simulink model "Temp"  (R2021a)
settings: Solver=FixedStepAuto  StartTime=0.0  StopTime=10.0  FixedStep=1e-3  RelTol=1e-3  EnableMultiTasking=on
undefined symbols (not defined in the file): D0, D10, D11, D12, D13, D2, D4, D5, D6, D7, D8, D9, PTA0, PTA2, PTB23, PTB9, PTC16, PTC2, PTC3, PTC4, PTD0, PTD1, PTD2, PTD3
libraries: frdmk64flib x16
settings Model: PacingRate=0.250000  ExtModeTrigDuration=5  Creator=Arun Mistry  LastModifiedBy=Arun Mistry
settings OptimizationCC: EnhancedBackFolding=on  PassReuseOutputArgsAs=Individual arguments  ZeroExternalMemoryAtStartup=off  ZeroInternalMemoryAtStartup=off  MaxStackSize=64  OptimizeBlockOrder=speed  DifferentSizesBufferReuse=on  OptimizationCustomize=off  EfficientTunableParamExpr=on
settings DebuggingCC: ParameterTunabilityLossMsg=error
settings HardwareCC: ProdBitPerPointer=32  ProdBitPerSizeT=32  ProdBitPerPtrDiffT=32  ProdLargestAtomicInteger=Long  ProdLargestAtomicFloat=Double  ProdWordSize=32  ProdHWDeviceType=ARM Compatible->ARM Cortex
settings SFSimCC: MATLABDynamicMemAlloc=off
settings RTWCC: SystemTargetFile=ert.tlc  HardwareBoard=NXP FRDM-K64F  TLCOptions="-aInlineSetEventsForThisBaseRateFcn=TLC_FALSE -aSuppressMultiTaskScheduler=TLC_FALSE  -aRateBasedStepFcn=0"  TemplateMakefile=ert_default_tmf  Toolchain=GNU Tools for ARM Embedded Processors
settings CodeAppCC: ForceParamTrailComments=on  IgnoreCustomStorageClasses=off  OperatorAnnotations=on  SimulinkDataObjDesc=on  SFDataObjDesc=on  InsertBlockDesc=on
settings ERTTargetCC: ExtModeTransport=4  ExtModeMexFile=sendToCommService

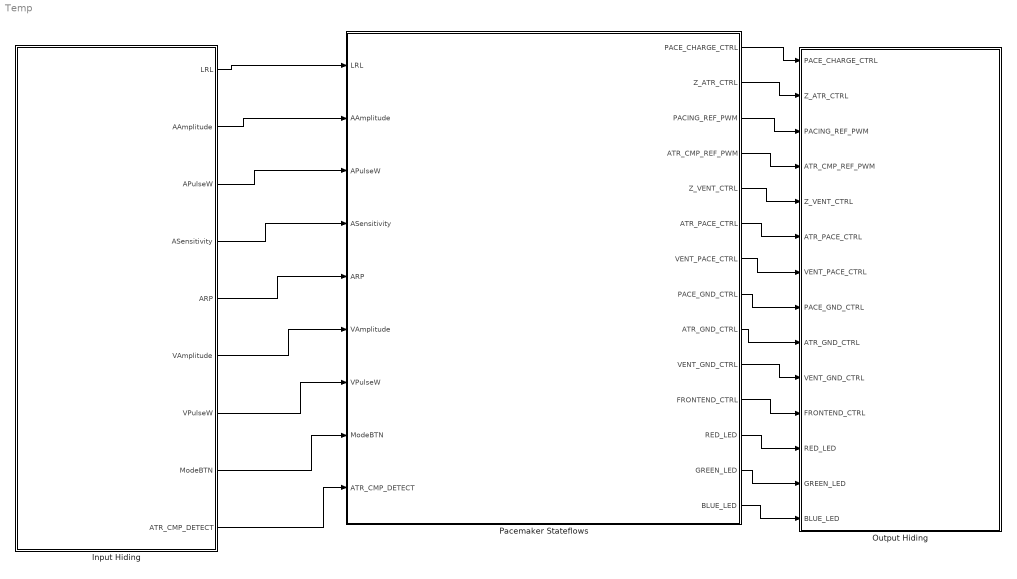
== system Temp ==
  Input Hiding : Subsystem
  Output Hiding : Subsystem
  Pacemaker Stateflows : Stateflow chart  TreatAsAtomicUnit=on
      settings: PortSchema="{\"entries\":[{\"content\":{\"sides\":[{\"content\":{\"connectorIds\":[\"In1\",\"In2\",\"In4\",\"In3\",\"In5\",\"In6\",\"In7\",\"In8\",\"In9\"]},\"type\":\"ConnectorPlacement.EquallySpacedRectSide\",\"uuid\":\"2299fccd-18a7-4758-b9fd-98bed0ea2d5f\"},{\"content\":{\"connectorIds\":[\"Out1\",\"Out2\",\"Out3\",\"Out4\",\"Out5\",\"Out6\",\"Out7\",\"Out8\",\"Out9\",\"Out10\",\"Out11\",\"Out12\",\"Out13\",\"Out14\"],\"side\":\"RIGHT\"},\"type\":\"ConnectorPlacement.EquallySpacedRectSide\",\"uuid\":\"a580a96d-c680-40ce-9bea-87ad4b87457c\"},{\"content\":{\"connectorIds\":[],\"side\":\"TOP\"},\"type\":\"ConnectorPlacement.EquallySpacedRectSide\",\"uuid\":\"b356f760-e5f1-4f6b-abb2-2757fd914320\"}]},\"type\":\"ConnectorPlacement.EquallySpacedConnector\",\"uuid\":\"b29a7396-67ba-49d5-b173-a751f9e05efc\"}],\"packageUris\":[\"http://schema.mathworks.com/mf0/Connector/R2020b\"],\"version\":\"1.0\"}"
  wires:
  Input Hiding/8(ModeBTN) -> Pacemaker Stateflows/8(ModeBTN)
  Input Hiding/2(AAmplitude) -> Pacemaker Stateflows/2(AAmplitude)
  Pacemaker Stateflows/2(Z_ATR_CTRL) -> Output Hiding/2(Z_ATR_CTRL)
  Pacemaker Stateflows/9(ATR_GND_CTRL) -> Output Hiding/9(ATR_GND_CTRL)
  Input Hiding/6(VAmplitude) -> Pacemaker Stateflows/6(VAmplitude)
  Pacemaker Stateflows/6(ATR_PACE_CTRL) -> Output Hiding/6(ATR_PACE_CTRL)
  Input Hiding/3(APulseW) -> Pacemaker Stateflows/4(APulseW)
  Pacemaker Stateflows/5(Z_VENT_CTRL) -> Output Hiding/5(Z_VENT_CTRL)
  Pacemaker Stateflows/3(PACING_REF_PWM) -> Output Hiding/3(PACING_REF_PWM)
  Pacemaker Stateflows/10(VENT_GND_CTRL) -> Output Hiding/10(VENT_GND_CTRL)
  Pacemaker Stateflows/8(PACE_GND_CTRL) -> Output Hiding/8(PACE_GND_CTRL)
  Pacemaker Stateflows/7(VENT_PACE_CTRL) -> Output Hiding/7(VENT_PACE_CTRL)
  Input Hiding/1(LRL) -> Pacemaker Stateflows/1(LRL)
  Input Hiding/7(VPulseW) -> Pacemaker Stateflows/7(VPulseW)
  Pacemaker Stateflows/1(PACE_CHARGE_CTRL) -> Output Hiding/1(PACE_CHARGE_CTRL)
  Input Hiding/4(ASensitivity) -> Pacemaker Stateflows/3(ASensitivity)
  Input Hiding/5(ARP) -> Pacemaker Stateflows/5(ARP)
  Input Hiding/9(ATR_CMP_DETECT) -> Pacemaker Stateflows/9(ATR_CMP_DETECT)
  Pacemaker Stateflows/12(RED_LED) -> Output Hiding/12(RED_LED)
  Pacemaker Stateflows/13(GREEN_LED) -> Output Hiding/13(GREEN_LED)
  Pacemaker Stateflows/11(FRONTEND_CTRL) -> Output Hiding/11(FRONTEND_CTRL)
  Pacemaker Stateflows/4(ATR_CMP_REF_PWM) -> Output Hiding/4(ATR_CMP_REF_PWM)
  Pacemaker Stateflows/14(BLUE_LED) -> Output Hiding/14(BLUE_LED)

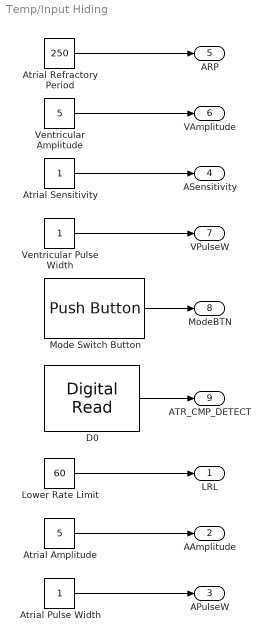
== system Temp/Input Hiding ==
  Atrial Amplitude : Constant  Value=5  OutDataTypeStr=double
  Atrial Pulse Width : Constant  OutDataTypeStr=double
  Atrial Refractory Period : Constant  Value=250  OutDataTypeStr=double
  Atrial Sensitivity : Constant  OutDataTypeStr=double
  D0 : frdmk64flib/Digital Read  Whichpin=PTC16 (D0)  SampleTime=-1
  Lower Rate Limit : Constant  Value=60  OutDataTypeStr=double
  Mode Switch Button : frdmk64flib/Push Button  Whichswitch=SW2  SampleTime1=-1
  Ventricular Amplitude : Constant  Value=5  OutDataTypeStr=double
  Ventricular Pulse Width : Constant  OutDataTypeStr=double
  LRL : Outport  OutDataTypeStr=double
  AAmplitude : Outport  Port=2  OutDataTypeStr=double
  APulseW : Outport  Port=3  OutDataTypeStr=double
  ASensitivity : Outport  Port=4  OutDataTypeStr=double
  ARP : Outport  Port=5  OutDataTypeStr=double
  VAmplitude : Outport  Port=6  OutDataTypeStr=double
  VPulseW : Outport  Port=7  OutDataTypeStr=double
  ModeBTN : Outport  Port=8  OutDataTypeStr=boolean
  ATR_CMP_DETECT : Outport  Port=9  OutDataTypeStr=boolean
  wires:
  Ventricular Amplitude/1 -> VAmplitude/1
  Mode Switch Button/1 -> ModeBTN/1
  D0/1 -> ATR_CMP_DETECT/1
  Atrial Refractory Period/1 -> ARP/1
  Ventricular Pulse Width/1 -> VPulseW/1
  Atrial Sensitivity/1 -> ASensitivity/1
  Atrial Pulse Width/1 -> APulseW/1
  Atrial Amplitude/1 -> AAmplitude/1
  Lower Rate Limit/1 -> LRL/1

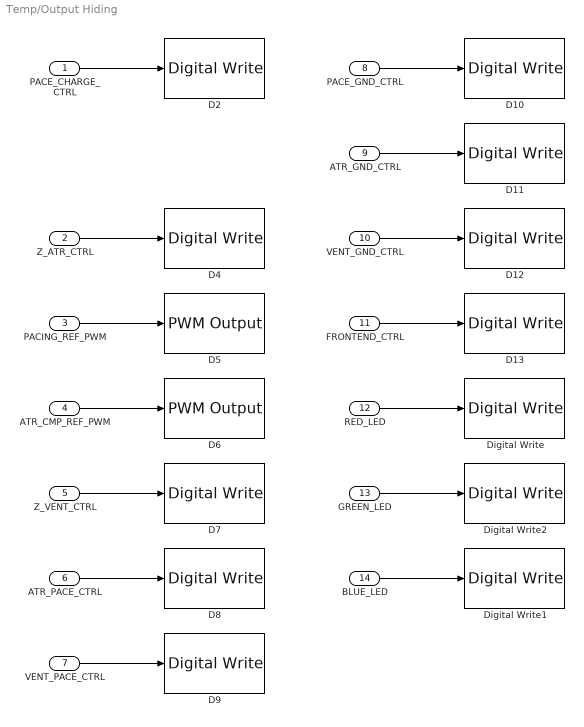
== system Temp/Output Hiding ==
  PACE_CHARGE_CTRL : Inport  OutDataTypeStr=double
  Z_ATR_CTRL : Inport  Port=2  OutDataTypeStr=double
  PACING_REF_PWM : Inport  Port=3  OutDataTypeStr=double
  ATR_CMP_REF_PWM : Inport  Port=4  OutDataTypeStr=double
  Z_VENT_CTRL : Inport  Port=5  OutDataTypeStr=double
  ATR_PACE_CTRL : Inport  Port=6  OutDataTypeStr=double
  VENT_PACE_CTRL : Inport  Port=7  OutDataTypeStr=double
  PACE_GND_CTRL : Inport  Port=8  OutDataTypeStr=double
  ATR_GND_CTRL : Inport  Port=9  OutDataTypeStr=double
  VENT_GND_CTRL : Inport  Port=10  OutDataTypeStr=double
  FRONTEND_CTRL : Inport  Port=11  OutDataTypeStr=double
  RED_LED : Inport  Port=12  OutDataTypeStr=double
  GREEN_LED : Inport  Port=13  OutDataTypeStr=double
  BLUE_LED : Inport  Port=14  OutDataTypeStr=double
  D10 : frdmk64flib/Digital Write  Whichpin=PTD0 (D10)
  D11 : frdmk64flib/Digital Write  Whichpin=PTD2 (D11)
  D12 : frdmk64flib/Digital Write  Whichpin=PTD3 (D12)
  D13 : frdmk64flib/Digital Write  Whichpin=PTD1 (D13)
  D2 : frdmk64flib/Digital Write  Whichpin=PTB9 (D2)
  D4 : frdmk64flib/Digital Write  Whichpin=PTB23 (D4)
  D5 : frdmk64flib/PWM Output  Whichpin=PTA2 (D5)  InitialFrequency=2000  InitialDutyCycle=100
  D6 : frdmk64flib/PWM Output  Whichpin=PTC2 (D6)  InitialFrequency=916  InitialDutyCycle=0
  D7 : frdmk64flib/Digital Write  Whichpin=PTC3 (D7)
  "D8 " : frdmk64flib/Digital Write  Whichpin=PTA0 (D8)
  D9 : frdmk64flib/Digital Write  Whichpin=PTC4 (D9)
  Digital Write : frdmk64flib/Digital Write  Whichpin=RED_LED
  Digital Write1 : frdmk64flib/Digital Write  Whichpin=BLUE_LED
  Digital Write2 : frdmk64flib/Digital Write  Whichpin=GREEN_LED
  wires:
  VENT_PACE_CTRL/1 -> D9/1
  ATR_CMP_REF_PWM/1 -> D6/1
  PACE_GND_CTRL/1 -> D10/1
  PACING_REF_PWM/1 -> D5/1
  ATR_GND_CTRL/1 -> D11/1
  ATR_PACE_CTRL/1 -> "D8 "/1
  PACE_CHARGE_CTRL/1 -> D2/1
  FRONTEND_CTRL/1 -> D13/1
  VENT_GND_CTRL/1 -> D12/1
  Z_ATR_CTRL/1 -> D4/1
  Z_VENT_CTRL/1 -> D7/1
  RED_LED/1 -> Digital Write/1
  GREEN_LED/1 -> Digital Write2/1
  BLUE_LED/1 -> Digital Write1/1

== stateflow chart Temp/Pacemaker Stateflows ==
  state AOO
    state ENTRY
      entry:
      VENT_PACE_CTRL = 0; VENT_GND_CTRL = 0; PACE_GND_CTRL = 1;
      Z_VENT_CTRL = 0; Z_ATR_CTRL = 0; PACING_REF_PWM = AAmplitude*20;
    state PACE_ATR
      entry:
      PACE_CHARGE_CTRL = 0;
      ATR_GND_CTRL = 0;
      ATR_PACE_CTRL = 1;
      RED_LED = 1;
    state C22_CHARGE
      entry:
      ATR_PACE_CTRL = 0;
      ATR_GND_CTRL = 1;
      PACE_CHARGE_CTRL = 1;
      RED_LED = 0;
    (default) -> AOO.ENTRY
    AOO.ENTRY -> AOO.C22_CHARGE
    AOO.PACE_ATR -> AOO.C22_CHARGE : after(APulseW,msec)
    AOO.C22_CHARGE -> AOO.PACE_ATR : after((60000/LRL)-APulseW,msec)
  state VOO
    state ENTRY
      entry:
      ATR_PACE_CTRL = 0; ATR_GND_CTRL = 0; PACE_GND_CTRL = 1;
      Z_ATR_CTRL = 0; Z_VENT_CTRL = 0; PACING_REF_PWM = VAmplitude*20;
    state PACE_VENT
      entry:
      PACE_CHARGE_CTRL = 0;
      VENT_GND_CTRL = 0;
      VENT_PACE_CTRL = 1;
      BLUE_LED = 1;
    state C22_CHARGE
      entry:
      VENT_PACE_CTRL = 0;
      VENT_GND_CTRL = 1;
      PACE_CHARGE_CTRL = 1;
      BLUE_LED = 0;
    (default) -> VOO.ENTRY
    VOO.ENTRY -> VOO.C22_CHARGE
    PACE_VENT -> VOO.C22_CHARGE : after(VPulseW,msec)
    VOO.C22_CHARGE -> PACE_VENT : after((60000/LRL)-VPulseW,msec)
  state MODE
    entry:
    Mode = Mode + 1;
    Mode = rem(Mode ,4);
  state AAI
    state ENTRY
      entry:
      VENT_PACE_CTRL = 0; VENT_GND_CTRL = 0; PACE_GND_CTRL = 1;
      Z_VENT_CTRL = 0; Z_ATR_CTRL = 0; PACING_REF_PWM = AAmplitude*20;
      FRONTEND_CTRL = 1;
    state PACE_ATR
      %Discharge
      entry:
      PACE_CHARGE_CTRL = 0;
      ATR_GND_CTRL = 0;
      ATR_PACE_CTRL = 1;
    state C22_CHARGE
      entry:
      ATR_PACE_CTRL = 0;
      ATR_GND_CTRL = 1;
      PACE_CHARGE_CTRL = 1;
    state INTERMEDIATE
      %In between state
      entry:
      PACE_CHARGE_CTRL = 1;
      ATR_GND_CTRL = 1;
      ATR_PACE_CTRL = 0;
    (default) -> AAI.ENTRY
    AAI.ENTRY -> AAI.C22_CHARGE
    AAI.C22_CHARGE -> AAI.PACE_ATR [order 1] : after((60000/LRL)-APulseW-ARP,msec)
    AAI.C22_CHARGE -> INTERMEDIATE [order 2] : [ATR_CMP_DETECT == true]{after(LRL,msec)}
    INTERMEDIATE -> AAI.C22_CHARGE : after(ARP,msec)
    AAI.PACE_ATR -> INTERMEDIATE : after(APulseW,msec)
  state VVI
    state ENTRY
      entry:
      VENT_PACE_CTRL = 0; VENT_GND_CTRL = 0; PACE_GND_CTRL = 1;
      Z_VENT_CTRL = 0; Z_ATR_CTRL = 0; FRONTEND_CTRL = 1;
      PACING_REF_PWM = AAmplitude*20; ATR_CMP_REF_PWM=ASensitivity/AAmplitude*100;
    state PACE_ATR
      %Discharge
      entry:
      PACE_CHARGE_CTRL = 0;
      ATR_GND_CTRL = 0;
      ATR_PACE_CTRL = 1;
      RED_LED = 1;
    state C22_CHARGE
      entry:
      ATR_PACE_CTRL = 0;
      ATR_GND_CTRL = 1;
      PACE_CHARGE_CTRL = 1;
      RED_LED = 0;
    state REFRACTORY
      entry:
      GREEN_LED = 1;
      exit:
      GREEN_LED = 0;
    (default) -> VVI.ENTRY
    VVI.ENTRY -> VVI.C22_CHARGE
    VVI.PACE_ATR -> VVI.C22_CHARGE : [after(APulseW,msec)]
    VVI.C22_CHARGE -> VVI.PACE_ATR [order 1] : after((60000/LRL)-APulseW,msec)
    VVI.C22_CHARGE -> REFRACTORY [order 2] : after(ARP,msec)[ATR_CMP_DETECT == true]
    REFRACTORY -> VVI.PACE_ATR [order 1] : after((60000/LRL)-ARP,msec)
    REFRACTORY -> REFRACTORY [order 2] : after(ARP,msec)[ATR_CMP_DETECT == true]
  (default) -> MODE
  MODE -> VOO [order 2] : [Mode==1&&ModeBTN==false]
  MODE -> AOO [order 1] : [Mode==0&&ModeBTN==false]
  VOO -> MODE : [ModeBTN==true]
  AOO -> MODE : [ModeBTN==true]
  MODE -> AAI [order 3] : [Mode==2&&ModeBTN==false]
  AAI -> MODE : [ModeBTN==true]
  VVI -> MODE : [ModeBTN==true]
  MODE -> VVI [order 4] : [Mode==3&&ModeBTN==false]
  data: LRL input double; AAmplitude input double; ASensitivity input; APulseW input double; ARP input; VAmplitude input double; VPulseW input double; PACE_CHARGE_CTRL output double; Z_ATR_CTRL output double; PACING_REF_PWM output double; ATR_CMP_REF_PWM output; Z_VENT_CTRL output double; ATR_PACE_CTRL output double; VENT_PACE_CTRL output double; PACE_GND_CTRL output double; ATR_GND_CTRL output double; VENT_GND_CTRL output double; FRONTEND_CTRL output; ModeBTN input boolean; Mode local double =1; ATR_CMP_DETECT input; RED_LED output; GREEN_LED output; BLUE_LED output
